simulink model "simple_FxTQESO"  (R2023a)
settings: Solver=ode1  StartTime=0.0  StopTime=60  FixedStep=0.01  RelTol=1e-3
values from neighbouring files (symbols this model uses):
  F = 5    [assignment3.m]
undefined symbols (not defined in the file or in its folder): Light, MIL
libraries: aerolibutil x8, sharedtransform x6, dspsrcs4 x6, sharedutil x3, simulink x2, matrix_library x1, robotcorelib x1, aerolibwind2 x1
settings Model: Creator=adan  LastModifiedBy=adan

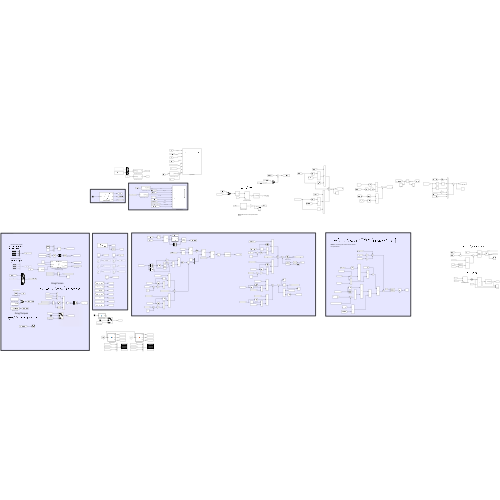
[thumbnail: Simulink's stored preview of the top-level diagram]
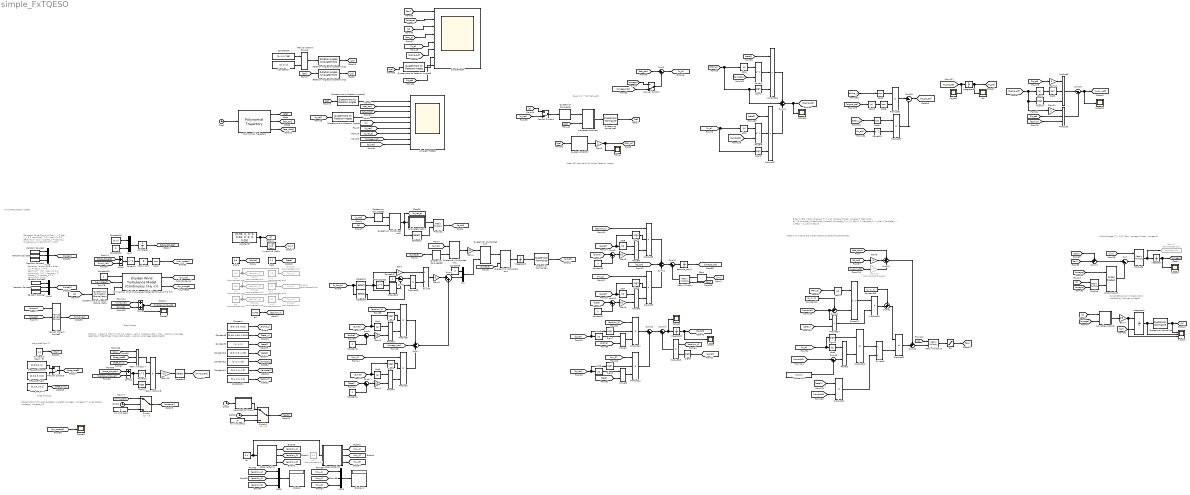
== system simple_FxTQESO ==
  note: $\frac{1}{2} \rho \alpha_{\eta} A_{\eta} (\omega - \omega_n)^ 2 \text{sign} (\omega - \omega_n)$
  note: Drag Torques
  note: $q_e = q^ *\otimes q_d$
  note: Note: PRV stands for Principal Rotation
      | Vector.
  note: $\tau = \Big [ \dot \omega_d + J^{-1} \omega \times J \omega + \frac{|\dot e|^{2-\lambda_2}\text{sign}(\dot e)}{\lambda_2 \xi_2} \Big (1 + \lambda_1 \xi_1|e|^{\lambda_1 - 1}\Big ) - u_{aux} \Big ]$
  note: Note: It is missing the Inertia Tensor outside
      | the parenthesis
  note: $\dot \omega = J^{-1} (\tau - \omega \times J \omega)$
  note: $\mathbf{\dot q} = \frac{1}{2} \mathbf{q} \otimes \omega$
  note: Gaussian Noise Signals
      | $\bar v_x = \bar v_y = 5 \text{ms}^{-1}, \bar v_z = 3 \text{ms}^{-1} \\ \sigma_x = \sigma_y = \sigma_z = 2 \text{ms}^{-1}$
  note: $\Delta _ {\eta} = \frac{1}{2}\rho \alpha _ \eta A _\eta\big (\dot d_\eta - \upsilon _{\omega \eta}\big)^2\text{sign }\big (\dot d_\eta - \upsilon _{\omega \eta}\big)$$
  note: Gaussian Noise Signals
      | $\bar v_x = \bar v_y = 6 \text{ms}^{-1}, \bar v_z = 2 \text{ms}^{-1} \\ \sigma_x = \sigma_y = \sigma_z = 2 \text{ms}^{-1}$
  note: drag coeff from []
  note: Drag Forces
  note: Wind Perturbation Model
  Abs{1..12} (12 alike) : Abs  SaturateOnIntegerOverflow=off
  Bias : Bias  Bias=[4, 0, 0; 0, -2, 0; 0, 0, 5]  SaturateOnIntegerOverflow=off
  Clock{,1..3} (4 alike) : Clock
  Constant : Constant  Value=[0.5; 0.5; 0.01]
  Constant{1,6..7,19} (4 alike) : Constant
  Constant10 : Constant  Value=[0.5; 0.5; 1.25]
  Constant11 : Constant  Value=[1.2; 1.2; 1.2]
  Constant12 : Constant  Value=[2; 2; 1.75]
  Constant13 : Constant  Value=[1; 1; 1]
  Constant14 : Constant  Value=[2;2;2]
  Constant15 : Constant  Value=[1; 1; 1]
  Constant16 : Constant  Value=[0; 0; 0.785]
  Constant17 : Constant  Value=[0; 0; 0]
  Constant18 : Constant  Value=[0; 0]
  Constant2 : Constant  Value=2
  Constant20 : Constant  Value=0
  Constant21 : Constant  Value=[0.4; 0.4; 0.2]
  Constant3 : Constant  Value=[0.05; 0.05; 0.001]
  Constant4 : Constant  Value=2
  Constant5 : Constant  Value=[0.03, 0, 0; 0, 0.03, 0; 0, 0, 0.05]
  Constant8 : Constant  Value=0
  Constant9 : Constant  Value=[ 1; 1; 1]
  Cross Product : matrix_library/Cross Product
  Display : Display
  Display1 : Display
  Divide : Product  Inputs=*/
  Divide3 : Product  Inputs=*/
  Gain{,2,11..12} (4 alike) : Gain  Gain=2
  Gain1 : Gain  Gain=1/3
  Gain10 : Gain  Gain=-0.5
  Gain13 : Gain  Commented=through  Gain=-1
  Gain3 : Gain  Gain=1/3
  Gain{4..7} (4 alike) : Gain  Gain=0.5
  Gain8 : Gain  Gain=-1
  Gain9 : Gain  Gain=0
  Goto11 : Goto  Commented=on  GotoTag=omega_dot
  Goto25 : Goto  Commented=on  GotoTag=epsilon_2
  Goto26 : Goto  Commented=on  GotoTag=epsilon_3
  Goto29 : Goto  Commented=on  GotoTag=mu_1
  Goto3 : Goto  Commented=on  GotoTag=epsilon_1
  Goto30 : Goto  Commented=on  GotoTag=mu_2
  Goto31 : Goto  Commented=on  GotoTag=mu_3
  Integrator : Integrator  InitialCondition=[0; 0; 0]
  Integrator1 : Integrator  InitialConditionSource=external
  Integrator2 : Integrator  InitialCondition=[0; 0; 0]
  Integrator3 : Integrator  InitialCondition="[0.9995    0.0252    0.0146   -0.0144]'"
  Integrator5 : Integrator  InitialCondition=[0;0;0]
  Invert 3x3 Matrix : aerolibutil/Invert  3x3 Matrix
  Kronecker product : Subsystem
      mask Display: image('$imagefile'); % Use "Edit Image" on toolstrip to change.
  Kronecker product4 : Subsystem
  Kt1 : Scope
  Kt_dot1 : Scope
  Lo : Constant  Value=3.1
  Lo1 : Constant  Commented=on  Value=3.9
  Manual Variant Source : simulink/Signal Routing/Manual Variant Source  NumChoices=2  LabelModeActiveChoice=V_2
  Manual Variant Source2 : simulink/Signal Routing/Manual Variant Source  NumChoices=3  LabelModeActiveChoice=V_1
  Manual Switch1 : ManualSwitch  CurrentSetting=0
  Manual Switch2 : ManualSwitch  CurrentSetting=0
  Manual Switch3 : ManualSwitch  CurrentSetting=0
  Matrix Sum : Sum  Inputs=+
  Matrix Multiply : Product  Multiplication=Matrix(*)
  Matrix Multiply5 : Product  Multiplication=Matrix(*)
  Matrix Multiply7 : Product  Inputs=3
  Matrix Multiply8 : Product  Inputs=3
  Mux : Mux  Inputs=2
  Mux{5..6,8..9} (4 alike) : Mux  Inputs=3
  Mux7 : Mux  Inputs=2
  PRV_e : Scope
  Polynomial Trajectory : robotcorelib/Polynomial Trajectory  WaypointSource=Internal  Waypoints=[0, 0, 0, 0, 0, 0; 0, 0, 0, 0, 0, 0; 0, 0, 1, 2.8, 4, 2.8]  TimePoints=[0, 12, 24, 36, 48, 60]  TimeInterval=[ 1, 4 ]  Method=Cubic Polynomial  ParameterSource=Internal  VelocityBoundaryCondition=zeros( 3, 6 )  AccelerationBoundaryCondition=zeros( 2, 5 )  SimulateUsing=Interpreted execution
  Power{1..9,12} (10 alike) : Math  Operator=pow
  Power10 : Math  Operator=square
  Power13 : Math  Operator=square
  Power14 : Math  Operator=square
  Product{,1..2,14} (4 alike) : Product  Multiplication=Matrix(*)
  Product{3..4,6..9,11..12,26..27} (10 alike) : Product  Inputs=3
  Product{13,15,20..24,29,31} (9 alike) : Product
  Quaternion Conjugate : aerolibutil/Quaternion Conjugate
  Quaternion Conjugate2 : aerolibutil/Quaternion Conjugate
  Quaternion Conjugate3 : aerolibutil/Quaternion Conjugate
  Quaternion Multiplication{2..5} (4 alike) : aerolibutil/Quaternion Multiplication
  Quaternion Normalize : sharedutil/Quaternion Normalize  aMode=aMode
  Quaternion Normalize1 : sharedutil/Quaternion Normalize  aMode=aMode
  Quaternion Normalize2 : sharedutil/Quaternion Normalize  aMode=aMode
  Quaternions to Direction Cosine Matrix : sharedtransform/Quaternions to  Direction Cosine Matrix  aMode=aMode
      settings: LibrarySourceBlock=|
      | aerolibtransform2/Quaternions to
      | Direction Cosine Matrix
  Quaternions to Rotation Angles : sharedtransform/Quaternions to Rotation Angles  rotationOrder=XYZ  aMode=aMode
  Quaternions to Rotation Angles1 : sharedtransform/Quaternions to Rotation Angles  rotationOrder=XYZ  aMode=aMode
  Quaternions to Rotation Angles2 : sharedtransform/Quaternions to Rotation Angles  rotationOrder=XYZ  aMode=aMode
  Random Source2 : dspsrcs4/Random Source  SrcType=Gaussian  NormMethod=Ziggurat  CltLength=12  MinVal=0  MaxVal=1  MeanVal=5  VarVal=2  RepMode=Not repeatable  rawSeed=1  IsInherit=off  SampMode=Discrete  SampTime=0.01  SampFrame=1  DataType=Double  OutComplex=Real  OutputFrames=off
  Random Source3 : dspsrcs4/Random Source  SrcType=Gaussian  NormMethod=Ziggurat  CltLength=12  MinVal=0  MaxVal=1  MeanVal=5  VarVal=2  RepMode=Not repeatable  rawSeed=1  IsInherit=off  SampMode=Discrete  SampTime=0.01  SampFrame=1  DataType=Double  OutComplex=Real  OutputFrames=off
  Random Source4 : dspsrcs4/Random Source  SrcType=Gaussian  NormMethod=Ziggurat  CltLength=12  MinVal=0  MaxVal=1  MeanVal=3  VarVal=2  RepMode=Not repeatable  rawSeed=1  IsInherit=off  SampMode=Discrete  SampTime=0.01  SampFrame=1  DataType=Double  OutComplex=Real  OutputFrames=off
  Random Source5 : dspsrcs4/Random Source  SrcType=Gaussian  NormMethod=Ziggurat  CltLength=12  MinVal=0  MaxVal=1  MeanVal=6  VarVal=2  RepMode=Not repeatable  rawSeed=1  IsInherit=off  SampMode=Discrete  SampTime=1  SampFrame=1  DataType=Double  OutComplex=Real  OutputFrames=off
  Random Source6 : dspsrcs4/Random Source  SrcType=Gaussian  NormMethod=Ziggurat  CltLength=12  MinVal=0  MaxVal=1  MeanVal=6  VarVal=2  RepMode=Not repeatable  rawSeed=1  IsInherit=off  SampMode=Discrete  SampTime=1  SampFrame=1  DataType=Double  OutComplex=Real  OutputFrames=off
  Random Source7 : dspsrcs4/Random Source  SrcType=Gaussian  NormMethod=Ziggurat  CltLength=12  MinVal=0  MaxVal=1  MeanVal=2  VarVal=2  RepMode=Not repeatable  rawSeed=1  IsInherit=off  SampMode=Discrete  SampTime=1  SampFrame=1  DataType=Double  OutComplex=Real  OutputFrames=off
  Rotation Angles to Quaternions1 : sharedtransform/Rotation Angles to Quaternions  rotationOrder=XYZ  aMode=aMode
  Rotation Angles to Quaternions2 : sharedtransform/Rotation Angles to Quaternions  rotationOrder=XYZ  aMode=aMode
  Scope{,1..3,7,10..11} (7 alike) : Scope
  Selector1 : Selector  InputPortWidth=4  IndexOptions=Index vector (dialog)  Indices=[2:4]  OutputSizes=1
  Selector4 : Selector  InputPortWidth=4  IndexOptions=Index vector (dialog)  Indices=[2:4]  OutputSizes=1
  Selector5 : Selector  InputPortWidth=4  IndexOptions=Index vector (dialog)  Indices=[1]  OutputSizes=1
  Selector8 : Selector  InputPortWidth=3  IndexOptions=Index vector (dialog)  Indices=[3]  OutputSizes=1
  Sign{1..12} (12 alike) : Signum
  Sqrt{1..2,4..6} (5 alike) : Sqrt
  Sum{,1,3,25} (4 alike) : Sum  Inputs=|+-
  Sum{4..6,9..10,12..14} (8 alike) : Sum  Inputs=|++
  Sum11 : Sum  Inputs=+++
  Sum15 : Sum  Inputs=+-
  Sum16 : Sum  Inputs=|--
  Sum17 : Sum  Inputs=++|
  Sum19 : Sum  Inputs=++-
  Sum2 : Sum  Inputs=+-
  Sum20 : Sum  Inputs=|-+
  Sum21 : Sum  Inputs=-+|
  Sum22 : Sum  Inputs=++|
  Sum23 : Sum  Inputs=++|
  Sum24 : Sum  Inputs=+++
  Sum7 : Sum  Inputs=+++
  Sum8 : Sum
  Switch : Switch  Criteria=u2 > Threshold  Threshold=5  SaturateOnIntegerOverflow=off  InputSameDT=off
  Switch1 : Switch  Criteria=u2 > Threshold  Threshold=5  SaturateOnIntegerOverflow=off  InputSameDT=off
  Transpose5 : Math  Operator=transpose
  Unit Delay : UnitDelay  SampleTime=0.01  HasFrameUpgradeWarning=on
  Von Karman Wind Turbulence Model (Continuous (+q +r)) : aerolibwind2/Dryden Wind Turbulence Model  (Continuous (+q -r))  units=Metric (MKS)  spec=MIL-F-8785C  model=Continuous Von Karman (+q +r)  W20=15  Wdeg=0  TurbProb=10^-2 - Light  L_high=762  Wingspan=10  ts=0.1  Seed=[23341 23342 23343 23344]  T_on=on
      settings: LibrarySourceBlock=|
      | aerolibwind2/Von Karman Wind Turbulence Model
      | (Continuous (+q +r))
  air density [kg/m^3] : Constant  Value=1.2
  alpha : Constant  Value=0.6
  area_per_axis : Constant  Value=[0.1;0.1;0.2]
  beta : Constant  Value=1.2
  calculateCvMatrix : MATLAB Function  TreatAsAtomicUnit=on
  drag_coeff_gus : Constant  Value=[0.3;0.3; 0.5]
  drag_coeff_paper : Constant  Value=[0.6;0.6; 1]
  e1 : Constant  Commented=on  Value=16
  e2 : Constant  Commented=on  Value=150
  e3 : Constant  Commented=on  Value=450
  e4 : Constant  Value=0.005
  gamma_hat_2 : Integrator  InitialCondition=[0; 0; 0]
  mu1 : Constant  Commented=on  Value=16
  mu2 : Constant  Commented=on  Value=20
  mu3 : Constant  Commented=on  Value=30
  no wind perb : Constant  Value=0
  no wind perb1 : Constant  Value=0
  observerGains : MATLAB Function  TreatAsAtomicUnit=on
  observerGains1 : MATLAB Function  TreatAsAtomicUnit=on
  perturbationTorque : MATLAB Function  TreatAsAtomicUnit=on
  q,q_dot : Scope  NumInputPorts=3
  quaterniontoPRV : Subsystem
  simpleFxTQESO : Scope  NumInputPorts=9
  simpleModel : Scope  NumInputPorts=8
  tau : Saturate
  wires:
  Clock/1 -> Polynomial Trajectory/1
  Polynomial Trajectory/3 -> [eta_ddot]
  Polynomial Trajectory/2 -> [eta_dot]
  Polynomial Trajectory/1 -> [eta]
  [q] -> simpleFxTQESO/5  "q"
  [q_hat] -> simpleFxTQESO/6  "q_hat"
  [eta_dot] -> simpleFxTQESO/2  "eta_dot"
  [q_hat_e] -> simpleFxTQESO/7  "q_hat_e"
  [q_hat] -> Quaternions to Rotation Angles/1
  Quaternions to Rotation Angles/1 -> simpleFxTQESO/4  "eta_hat"
  Constant5/1 -> Invert 3x3 Matrix/1, [J]
  Invert 3x3 Matrix/1 -> [Jinv]
  [td_hat] -> simpleFxTQESO/9  "Td_hat"
  [omega_hat] -> simpleFxTQESO/8  "omega_hat"
  [eta_ddot] -> simpleFxTQESO/3
  Transpose5/1 -> Product14/1
  Product14/1 -> Sum3/2
  Constant7/1 -> Sum3/1
  Sum3/1 -> Product15/1
  Selector5/1 -> Product15/2
  Sum4/1 -> Mux/2
  Constant8/1 -> Mux/1
  [q_hat_e] -> Quaternion Conjugate3/1
  [q_hat] -> Quaternion Multiplication2/1
  Mux/1 -> Quaternion Multiplication3/2
  [q_hat_e] -> Quaternion Multiplication4/2
  Quaternion Multiplication3/1 -> Quaternion Multiplication4/1
  Quaternion Multiplication4/1 -> Integrator3/1
  Integrator3/1 -> Quaternion Normalize1/1
  Quaternion Normalize1/1 -> [q_hat]
  Quaternion Conjugate2/1 -> Quaternion Multiplication5/1
  [q_hat] -> Quaternion Conjugate2/1
  Quaternion Multiplication5/1 -> Selector1/1, calculateCvMatrix/1(q), [q_hat_e]
  [q] -> Quaternion Multiplication5/2
  Quaternion Multiplication2/1 -> Gain4/1
  Quaternion Conjugate3/1 -> Quaternion Multiplication2/2
  Gain4/1 -> Quaternion Multiplication3/1
  calculateCvMatrix/1(Cv) -> Product1/1
  Selector1/1 -> Product1/2
  Product1/1 -> [e_hat]
  [q_hat_e] -> Selector5/1, Selector4/1
  Selector4/1 -> Gain/1, Product14/2, Transpose5/1
  Product15/1 -> Divide/2
  Gain/1 -> Divide/1
  alpha/1 -> [alpha]
  e2/1 -> Goto30/1, Goto25/1
  e3/1 -> Goto31/1, Goto26/1
  e4/1 -> [epsilon_4]
  beta/1 -> [beta]
  e1/1 -> Goto29/1, Goto3/1
  Sum6/1 -> Gain1/1
  Gain3/1 -> Power3/2
  [e_hat] -> Sign4/1, Abs5/1
  Abs5/1 -> Power4/1
  Power3/1 -> Product6/3
  [epsilon_1] -> Product6/1
  [e_hat] -> Sign3/1, Abs4/1
  [alpha] -> Sum5/1
  Power4/1 -> Product7/3
  [beta] -> Sum6/1
  Sign4/1 -> Product7/2
  [mu_1] -> Product7/1
  Abs4/1 -> Power3/1
  Constant2/1 -> Sum5/2
  Product7/1 -> Sum7/3
  Gain1/1 -> Power4/2
  [omega_hat] -> Sum7/2
  Constant4/1 -> Sum6/2
  Sum5/1 -> Gain3/1
  Sign3/1 -> Product6/2
  Product6/1 -> Sum7/1
  Divide/1 -> Gain9/1
  Sum7/1 -> Sum4/2
  Sum11/1 -> Sum12/1
  Constant6/1 -> Sum9/2
  Power5/1 -> Product8/3
  Product8/1 -> Sum11/1
  Sign7/1 -> Product11/2
  gamma_hat_2/1 -> [omega_hat]  "gamma_hat_2"
  Product13/1 -> Sum14/2
  Abs7/1 -> Power6/1
  [alpha] -> Power7/2
  Sign6/1 -> Product9/2
  [alpha] -> Sum9/1
  Product12/1 -> Sum13/2
  Sum13/1 -> Sum14/1
  Sum10/1 -> Gain6/1
  [e_hat] -> Sign5/1, Abs6/1
  [e_hat] -> Sign9/1
  Sign5/1 -> Product8/2
  Sum9/1 -> Gain5/1
  [epsilon_3] -> Product11/1
  [mu_3] -> Product12/1
  Product9/1 -> Sum11/3
  [epsilon_2] -> Product8/1
  Power8/1 -> Product12/3
  [mu_2] -> Product9/1
  [beta] -> Sum10/1
  Abs9/1 -> Power8/1
  [e_hat] -> Sign6/1, Abs7/1
  Gain5/1 -> Power5/2
  Power6/1 -> Product9/3
  Gain6/1 -> Power6/2
  Sign8/1 -> Product12/2
  Sum12/1 -> gamma_hat_2/1
  [epsilon_4] -> Product13/1
  Integrator2/1 -> Scope/1, [td_hat]
  Abs8/1 -> Power7/1
  Product11/1 -> Sum13/1
  Abs6/1 -> Power5/1
  [e_hat] -> Abs8/1, Sign7/1
  Constant1/1 -> Sum10/2
  Sign9/1 -> Product13/2
  Power7/1 -> Product11/3
  [e_hat] -> Abs9/1, Sign8/1
  Sum14/1 -> Scope1/1, Integrator2/1
  [td_hat] -> Sum11/2
  [beta] -> Power8/2
  Quaternion Normalize2/1 -> [qe]  "qe"
  Gain2/1 -> PRV_e/1, [PRV_e]  "PRV_e"
  Kronecker product4/1(r) -> Quaternion Normalize2/1  "qe"
  quaterniontoPRV/1(lnq) -> Gain2/1
  [qe] -> quaterniontoPRV/1(q)
  [q] -> Manual Switch2/1
  [qd] -> Kronecker product4/2(p)
  Quaternion Conjugate/1 -> Kronecker product4/1(q)
  [eta] -> Rotation Angles to Quaternions1/1
  Rotation Angles to Quaternions1/1 -> [qd]
  Constant/1 -> [alpha_u]
  Constant3/1 -> [beta_u]
  Power1/1 -> Product26/2
  [w_e] -> Abs2/1, Sign2/1
  [zeta1] -> Product26/1
  Abs2/1 -> Power9/1
  Power9/1 -> Product27/2
  Sign2/1 -> Product27/3
  [PRV_e] -> Sum24/2, Sign1/1, Abs1/1
  [zeta2] -> Product27/1
  [lambda2] -> Power9/2
  Abs1/1 -> Power1/1
  Product26/1 -> Sum24/1
  Product27/1 -> Sum24/3
  Sum24/1 -> Scope10/1, [sigma_att]  "sigma_att"
  [lambda1] -> Power1/2
  Sign1/1 -> Product26/3
  [Kt_dot_att] -> Kt_dot1/1, Integrator5/1
  Product29/1 -> Sum25/2
  Product31/1 -> Sum25/1
  Sqrt4/1 -> Product29/1
  Abs10/1 -> Sqrt6/1
  Sqrt5/1 -> Product31/1
  Sqrt6/1 -> Product31/2
  Power10/1 -> Product29/2
  Integrator5/1 -> Kt1/1, [Kt_att]  "Kt_att"
  [Kt_att] -> Power10/1
  [beta_u] -> Sqrt4/1
  Sum25/1 -> [Kt_dot_att]
  [sigma_att] -> Abs10/1
  [alpha_u] -> Sqrt5/1
  Constant9/1 -> [zeta1]
  Constant10/1 -> [zeta2]
  Constant12/1 -> [lambda1]
  Constant11/1 -> [lambda2]
  tau/1 -> [tau]  "tau"
  Power2/1 -> Product20/2
  Sum20/1 -> Power2/2
  Product22/1 -> Sum23/2
  Sum22/1 -> Product22/1
  Sum21/1 -> Power12/2
  Gain8/1 -> Sum19/2
  Power12/1 -> Product23/1
  [u_aux_att] -> Gain13/1
  Sign11/1 -> Product20/1
  [lambda2] -> Sum20/1
  [PRV_e] -> Abs12/1
  Constant13/1 -> Sum21/1
  [lambda2] -> Product21/2
  Abs12/1 -> Power12/1
  [w_e] -> Sign11/1, Abs3/1
  Product20/1 -> Divide3/1
  [zeta1] -> Product24/2
  [zeta2] -> Product21/1
  Constant14/1 -> Sum20/2
  Matrix Multiply5/1 -> tau/1
  Product21/1 -> Divide3/2
  [lambda1] -> Product24/1, Sum21/2
  Product23/1 -> Sum22/2
  Product24/1 -> Product23/2
  [J] -> Matrix Multiply5/1
  [eta_ddot] -> Sum19/1
  Abs3/1 -> Power2/1
  Constant15/1 -> Sum22/1
  Divide3/1 -> Product22/2
  Sum23/1 -> Matrix Multiply5/2
  Product2/1 -> Goto11/1, Integrator/1
  Cross Product/1 -> Sum/2
  [omega] -> Cross Product/1
  [Jinv] -> Product2/1
  [omega] -> Kronecker product/2(p)
  [omega] -> Product/2
  Quaternion Normalize/1 -> q,q_dot/1, [q]  "q"
  Integrator/1 -> Scope7/1, [omega]  "omega"
  Product/1 -> Cross Product/2
  [J] -> Product/1
  [tau] -> Sum17/2
  [q0] -> Integrator1/2
  [q] -> Kronecker product/1(q)
  Gain7/1 -> q,q_dot/3, Integrator1/1
  Integrator1/1 -> q,q_dot/2, Quaternion Normalize/1
  Kronecker product/1(r) -> Gain7/1
  Sum/1 -> Product2/2
  Constant16/1 -> Manual Variant Source/1
  Rotation Angles to Quaternions2/1 -> [q0]
  [eta_dot] -> Sum1/1
  [omega] -> Manual Switch1/1
  Sum1/1 -> [w_e]
  [omega] -> simpleModel/2  "omega_"
  [tau] -> simpleModel/1  "torque"
  [q] -> simpleModel/3  "q"
  [w_e] -> simpleModel/5  "w_e"
  [PRV_e] -> simpleModel/4  "prv_e"
  Matrix Multiply/1 -> Sum12/2
  [Jinv] -> Bias/1
  [tau] -> Matrix Multiply/2
  Sum19/1 -> Sum23/1
  [td_hat] -> Gain8/1
  Manual Switch1/1 -> Sum1/2
  Manual Switch2/1 -> Quaternion Conjugate/1
  [q_hat] -> Manual Switch2/2
  [omega_hat] -> Manual Switch1/2
  Gain9/1 -> Sum4/1
  Manual Variant Source/1 -> Rotation Angles to Quaternions2/1
  Constant17/1 -> Manual Variant Source/2
  Constant18/1 -> Mux7/1
  Clock3/1 -> Switch/2
  Power13/1 -> Matrix Multiply8/2
  drag_coeff_gus/1 -> Manual Switch3/2
  [wind_vel] -> Sum8/1
  drag_coeff_paper/1 -> Manual Switch3/1
  Selector8/1 -> [Wind_perb]  "wind_perb"
  [Wind_perb] -> Switch/1
  Random Source5/1 -> Mux6/1
  Manual Variant Source2/1 -> [wind_vel]
  Constant19/1 -> Von Karman Wind Turbulence Model (Continuous (+q +r))/1
  Unit Delay/1 -> [pose_dot_eta]
  Matrix Multiply8/1 -> Gain10/1
  [pose_dot_eta] -> Sum15/1
  no wind perb/1 -> Switch/3
  Matrix Sum/1 -> Sqrt1/1
  Von Karman Wind Turbulence Model (Continuous (+q +r))/1 -> [tur_vel]
  Mux5/1 -> [noise1]
  Matrix Multiply7/1 -> Matrix Multiply8/1
  Random Source7/1 -> Mux6/3
  [rho] -> Matrix Multiply7/1
  Random Source2/1 -> Mux5/1
  [noise1] -> Manual Variant Source2/1
  [area_axis] -> Matrix Multiply7/3
  Mux7/1 -> Unit Delay/1
  Sum15/1 -> Sign12/1, Power13/1
  [pose_dot_eta] -> Sum2/1
  area_per_axis/1 -> [area_axis]
  [q] -> Quaternions to Direction Cosine Matrix/1
  Sum8/1 -> Scope2/1, [inertial_wind_vel]
  Switch/1 -> [external]
  Sum2/1 -> Power14/1
  Quaternions to Direction Cosine Matrix/1 -> Von Karman Wind Turbulence Model (Continuous (+q +r))/3
  [tur_vel] -> Sum8/2
  Sign12/1 -> Matrix Multiply8/3
  [noise2] -> Manual Variant Source2/2
  Mux6/1 -> [noise2]
  Random Source3/1 -> Mux5/2
  air density [kg/m^3]/1 -> [rho]
  Random Source4/1 -> Mux5/3
  Manual Switch3/1 -> [drag_coeff]
  [wind_vel] -> Sum2/2
  Constant20/1 -> Mux7/2
  [uav_speed] -> Von Karman Wind Turbulence Model (Continuous (+q +r))/2
  Gain10/1 -> Selector8/1  "wind_perb"
  [inertial_wind_vel] -> Sum15/2
  [drag_coeff] -> Matrix Multiply7/2
  Power14/1 -> Matrix Sum/1
  Random Source6/1 -> Mux6/2
  Sqrt1/1 -> [uav_speed]  "uav_speed"
  Von Karman Wind Turbulence Model (Continuous (+q +r))/2 -> [tur_omega]
  [Kt_att] -> Gain12/1
  Product4/1 -> Sum16/2
  [epsilon] -> Product4/3
  [Kt_att] -> Product4/2
  Abs11/1 -> Sqrt2/1
  Product3/1 -> Sum16/1
  Sqrt2/1 -> Product3/2
  Gain11/1 -> Product4/1
  Sign10/1 -> Product3/3
  Gain12/1 -> Product3/1
  [sigma_att] -> Abs11/1, Gain11/1, Sign10/1
  Constant21/1 -> [epsilon]
  Quaternions to Rotation Angles1/1 -> simpleFxTQESO/1  "eta_d"
  [qd] -> Quaternions to Rotation Angles1/1
  Sum16/1 -> Scope11/1, [u_aux_att]
  Sum17/1 -> Sum/1
  [perb] -> Sum17/1
  Clock1/1 -> perturbationTorque/1(t)
  perturbationTorque/1(td) -> Switch1/1
  [tur_omega] -> Scope3/1
  [sigma_att] -> simpleModel/6
  [qe] -> Quaternions to Rotation Angles2/1
  Quaternions to Rotation Angles2/1 -> simpleModel/7  "eta_e"
  Gain13/1 -> Sum19/3
  observerGains/1(K1) -> [epsilon_1]
  observerGains/2(K2) -> [epsilon_2]
  observerGains/3(K3) -> [epsilon_3]
  Lo/1 -> observerGains1/1(Lo), observerGains/1(Lo)
  [epsilon_3] -> Mux8/3
  [epsilon_2] -> Mux8/2
  [epsilon_1] -> Mux8/1
  Mux8/1 -> Display/1
  observerGains1/3(K3) -> [mu_3]
  observerGains1/2(K2) -> [mu_2]
  observerGains1/1(K1) -> [mu_1]
  [mu_1] -> Mux9/1
  [mu_2] -> Mux9/2
  Mux9/1 -> Display1/1
  [mu_3] -> Mux9/3
  Clock2/1 -> Switch1/2
  no wind perb1/1 -> Switch1/3
  Switch1/1 -> [perb]
  Bias/1 -> Matrix Multiply/1
  [Kt_att] -> simpleModel/8

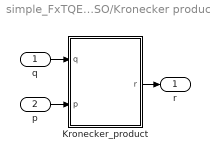
== system simple_FxTQESO/Kronecker product ==
  q : Inport
  p : Inport  Port=2
  Kronecker_product : MATLAB Function  TreatAsAtomicUnit=on
  r : Outport
  wires:
  q/1 -> Kronecker_product/1(q)
  p/1 -> Kronecker_product/2(p)
  Kronecker_product/1(r) -> r/1

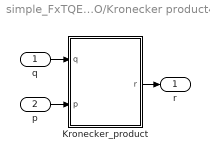
== system simple_FxTQESO/Kronecker product4 ==
  q : Inport
  p : Inport  Port=2
  Kronecker_product : MATLAB Function  TreatAsAtomicUnit=on
  r : Outport
  wires:
  q/1 -> Kronecker_product/1(q)
  p/1 -> Kronecker_product/2(p)
  Kronecker_product/1(r) -> r/1

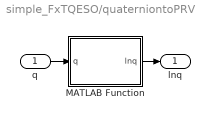
== system simple_FxTQESO/quaterniontoPRV ==
  q : Inport
  MATLAB Function : MATLAB Function  TreatAsAtomicUnit=on
  lnq : Outport
  wires:
  MATLAB Function/1(lnq) -> lnq/1
  q/1 -> MATLAB Function/1(q)

== matlab function simple_FxTQESO/Kronecker product/Kronecker_product ==
  data: q input; r output size=[4 1]; p input
function r = fcn(q, p)

%{
    Function to describe in matrix math the Kronecker product between
    two quaternions
    
    r = p kronecker q
    %}

    len = length(p);

    if len == 3 && length(q) == 4
        p1 = [0; p];
        q0 = q(1);
        q1 = q(2);
        q2 = q(3);
        q3 = q(4);
        
        % skew symmetric matrix
        q_matrix = [q0, -q1, -q2, -q3;
                  q1, q0, -q3, q2;
                  q2, q3, q0, -q1;
                  q3, -q2, q1, q0];
        
        r = q_matrix * p1;

    elseif len == 4
        q0 = q(1);
        q1 = q(2);
        q2 = q(3);
        q3 = q(4);
        
        % skew symmetric matrix
        q_matrix = [q0, -q1, -q2, -q3;
                  q1, q0, -q3, q2;
                  q2, q3, q0, -q1;
                  q3, -q2, q1, q0];
        
        r = q_matrix * p;

    else
        error('Quaternions dimensions do not match')
    end

== matlab function simple_FxTQESO/observerGains ==
  data: Lo input; K1 output; K2 output; K3 output
function [K1, K2, K3] = fcn(Lo)

K1 = 3 * Lo ^ (5/3);

K2 = 2 * Lo ^ (10/3);

K3 = (4/9) * Lo ^ (5);

== matlab function simple_FxTQESO/observerGains1 ==
  data: Lo input; K1 output; K2 output; K3 output
function [K1, K2, K3] = fcn(Lo)

K1 = 3 * Lo ^ (5/3);

K2 = 2 * Lo ^ (10/3);

K3 = (4/9) * Lo ^ (5);

== matlab function simple_FxTQESO/calculateCvMatrix ==
  data: q input; Cv output
function Cv = fcn(q)

q0 = q(1);
q1 = q(2);
q2 = q(3);
q3 = q(4);

Cv = [q0, -q3, q2;
      q3, q0, -q1;
      -q2, q1, q0] * 0.5;

Cv = pinv(Cv);

== matlab function simple_FxTQESO/quaterniontoPRV/MATLAB Function ==
  data: q input; lnq output size=[3 1]
function lnq = fcn(q)

if length(q) == 4
    q0 = q(1);
    q_vec = [q(2); q(3); q(4)];

    if norm(q_vec) == 0
        lnq = [0; 0; 0];
    else
        % q0 = real(q0);
        lnq = (q_vec / (norm(q_vec)) ) * acos(q0);
    end
else
    error('Input must be a vector 4 by 1 (Quaternion)')
end

== matlab function simple_FxTQESO/Kronecker product4/Kronecker_product ==
  data: q input; r output size=[4 1]; p input
function r = fcn(q, p)

%{
    Function to describe in matrix math the Kronecker product between
    two quaternions
    
    r = p kronecker q
    %}

    len = length(p);

    if len == 3 && length(q) == 4
        p1 = [0; p];
        q0 = q(1);
        q1 = q(2);
        q2 = q(3);
        q3 = q(4);
        
        % skew symmetric matrix
        q_matrix = [q0, -q1, -q2, -q3;
                  q1, q0, -q3, q2;
                  q2, q3, q0, -q1;
                  q3, -q2, q1, q0];
        
        r = q_matrix * p1;

    elseif len == 4
        q0 = q(1);
        q1 = q(2);
        q2 = q(3);
        q3 = q(4);
        
        % skew symmetric matrix
        q_matrix = [q0, -q1, -q2, -q3;
                  q1, q0, -q3, q2;
                  q2, q3, q0, -q1;
                  q3, -q2, q1, q0];
        
        r = q_matrix * p;

    else
        error('Quaternions dimensions do not match')
    end

== matlab function simple_FxTQESO/perturbationTorque ==
  data: t input; td output
function td = fcn(t)

td = [0.002 * sin(0.1 * t);
      0.0025 * sin(0.12 * t);
      0.005 * sin(0.2 * t)];
